simulink model "bldc_normal"  (R2020b)
settings: Solver=ode23t  StartTime=0  StopTime=500  FixedStep=Ts  MaxStep=1e-6  RelTol=1e-6  AbsTol=1e-6  EnableMultiTasking=on
PreLoadFcn:
  | assignin('base','Ts',[5e-6])
values from neighbouring files (symbols this model uses):
  N = speed.signals.values    [code.m]
libraries: powerlib x14
Description:
  | This demonstration illustrates use of the BLDC in a closed-loop
  | speed and voltage control on a 1 kW, 3000 rpm industrial motor
  | 
  | 
  | Copyright 2008-2010 The MathWorks, Inc.
settings Model: ExtModeAutoUpdateStatusClock=off  Creator=MathWorks  LastModifiedBy=yuvan
settings SolverCC: AutoScaleAbsTol=off  ZeroCrossControl=DisableAll  ZeroCrossAlgorithm=Adaptive
settings DataIOCC: LimitDataPoints=on  SaveFormat=Array  SignalLoggingSaveFormat=ModelDataLogs  ReturnWorkspaceOutputs=off  SignalLoggingName=sigsOut
settings OptimizationCC: ExpressionDepthLimit=2147483647  InitFltsAndDblsToZero=on  LifeSpan=inf
settings DebuggingCC: UnderspecifiedInitializationDetection=Classic  MergeDetectMultiDrivingBlocksExec=none  SignalResolutionControl=TryResolveAllWithWarning  MultiTaskDSMMsg=warning  MultiTaskCondExecSysMsg=none  FcnCallInpInsideContextMsg=warning  StateNameClashWarn=warning  SFUnexpectedBacktrackingDiag=warning  SFNoUnconditionalDefaultTransitionDiag=warning  SFExecutionAtInitializationDiag=none  ArithmeticOperatorsInVariantConditions=warning
settings HardwareCC: ProdBitPerPointer=32  ProdBitPerSizeT=32  ProdBitPerPtrDiffT=32  ProdLargestAtomicFloat=None  ProdIntDivRoundTo=Undefined  ProdEndianess=Unspecified  ProdWordSize=32  ProdHWDeviceType=32-bit Generic  TargetUnknown=on
settings ModelReferenceCC: PropagateSignalLabelsOutOfModel=off
settings SFSimCC: SimUseLocalCustomCode=off  CustomCodeUndefinedFunction=UseInterfaceOnly
settings RTWCC: RTWUseLocalCustomCode=off
settings CodeAppCC: StateflowObjectComments=on
settings GRTTargetCC: TargetLangStandard=C89/C90 (ANSI)  CombineOutputUpdateFcns=off  GRTInterface=on
settings ConfigComp: CovMetricSettings=dw  CovSaveCumulativeToWorkspaceVar=on  CovSaveSingleToWorkspaceVar=on  CovExternalEMLEnable=off
settings SimscapeCC: SimscapeNormalizeSystem=off

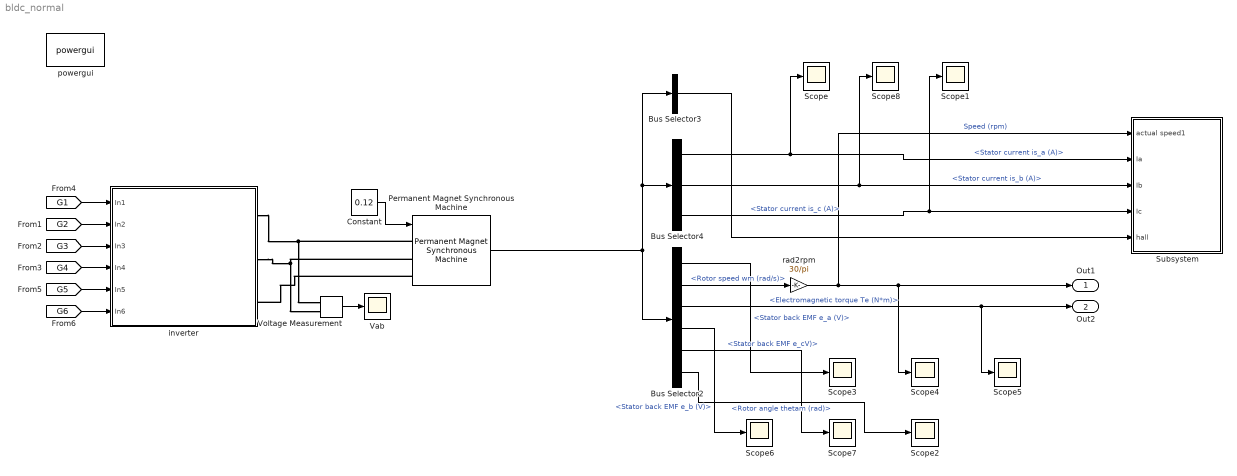
== system bldc_normal ==
  Bus Selector2 : BusSelector  OutputSignals=Stator back EMF e_a (V),Rotor speed wm (rad/s),Electromagnetic torque Te (N*m),Stator back EMF e_b (V),Stator back EMF e_cV),Rotor angle thetam (rad)
  Bus Selector3 : BusSelector  OutputSignals=Hall effect signal h_a,Hall effect signal h_b,Hall effect signal h_c  OutputAsBus=on
  Bus Selector4 : BusSelector  OutputSignals=Stator current is_a (A),Stator current is_b (A),Stator current is_c (A)
  Constant : Constant  Value=0.12
  Permanent Magnet Synchronous Machine : powerlib/Machines/Permanent Magnet Synchronous Machine  NbPhases=3  FluxDistribution=Trapezoidal  RotorType=Round  MechanicalLoad=Torque Tm  PresetModel=No  ShowDetailedParameters=on  MeasurementBus=off  Resistance=0.18  Inductance=0.000835  dqInductances=[8.5e-3,8.5e-3]  La=0.000835  MachineConstant=Torque Constant (N.m / A_peak)  Flux=0.015  VoltageCst=12.5664  TorqueCst=0.12  Flat=120  Mechanical=[0.000621417 0.000303448 4]  PolePairs=4  InitialConditions=[0,0, 0,0]  InitialConditions5ph=[0 0 0 0 0 0]  RefAngle=90 degrees behind phase A axis (modified Park)  IterativeDiscreteModel=Trapezoidal non iterative  TsBlock=-1  TsPowergui=0
  Scope{,1..8} (9 alike) : Scope
  Subsystem : Subsystem
  Vab : Scope
  Voltage Measurement : powerlib/Measurements/Voltage Measurement  PhasorSimulation=off  OutputType=Complex  PSBequivalent=0
  inverter : Subsystem
  powergui : powerlib/powergui  Priority=1  SimulationMode=Continuous  SampleTime=5e-6  frequency=60  Iterations=50  frequencyindice=0  Pbase=100e6  ErrMax=1e-4  UnitsV=kV  UnitsW=MW  buscounter=0  FunctionMessages=off  echomessages=off  EnableUseOfTLC=off  CurrentSourceSwitches=on  DisableSnubberDevices=off  DisableRonSwitches=off  DisableVfSwitches=off  DisplayEquations=off  AutomaticDiscreteSolvers=off  SolverType=Tustin/Backward Euler (TBE)  Interpol=off  ExternalGateDelay=off  methode=off  Ts=100  x0status=blocks  SPID=off  SwTol=0  HookPort=off  NonlinearTolerance=1e-4  nMaxIteration=100  ContinueOnMaxIteration=off  RestoreLinks=warning  ResistiveCurrentMeasurement=off  Frange=[0:2:500]  Ylog=off  Xlog=on  ShowGrid=off  save=off  variable=ZData  structure=0  ZoomFFT=off  StartTime=0.0  cycles=1  DisplayStyle=1  fundamental=60  FreqAxis=off  MaxFrequency=1000  frequencyindicesteady=1  RmsSteady=1  display=off
  rad2rpm : Gain  Gain=30/pi
  Out1 : Outport  VectorParamsAs1DForOutWhenUnconnected=off
  Out2 : Outport  Port=2  VectorParamsAs1DForOutWhenUnconnected=off
  wires:
  Constant/1 -> Permanent Magnet Synchronous Machine/1
  Voltage Measurement/1 -> Vab/1
  Permanent Magnet Synchronous Machine/1 -> Bus Selector3/1, Bus Selector4/1, Bus Selector2/1
  Bus Selector2/3 -> Scope5/1, Out2/1  "<Electromagnetic torque Te (N*m)>"
  rad2rpm/1 -> Subsystem/1(actual speed1), Scope4/1, Out1/1  "Speed (rpm)"
  Bus Selector2/2 -> rad2rpm/1  "<Rotor speed wm (rad/s)>"
  Bus Selector3/1 -> Subsystem/5(hall)
  Bus Selector4/1 -> Scope/1, Subsystem/2(Ia)  "<Stator current is_a (A)>"
  Bus Selector4/2 -> Scope8/1, Subsystem/3(Ib)  "<Stator current is_b (A)>"
  Bus Selector4/3 -> Scope1/1, Subsystem/4(Ic)  "<Stator current is_c (A)>"
  [G1] -> inverter/1(In1)
  [G2] -> inverter/2(In2)
  [G3] -> inverter/3(In3)
  [G4] -> inverter/4(In4)
  [G5] -> inverter/5(In5)
  [G6] -> inverter/6(In6)
  Bus Selector2/4 -> Scope6/1  "<Stator back EMF e_b (V)>"
  Bus Selector2/5 -> Scope7/1  "<Stator back EMF e_cV)>"
  Bus Selector2/6 -> Scope2/1  "<Rotor angle thetam (rad)>"
  Bus Selector2/1 -> Scope3/1  "<Stator back EMF e_a (V)>"
  connections:
  Permanent Magnet Synchronous Machine/LConn3 -- inverter/RConn3
  inverter/RConn1 -- Permanent Magnet Synchronous Machine/LConn1 -- Voltage Measurement/LConn1
  inverter/RConn2 -- Permanent Magnet Synchronous Machine/LConn2 -- Voltage Measurement/LConn2

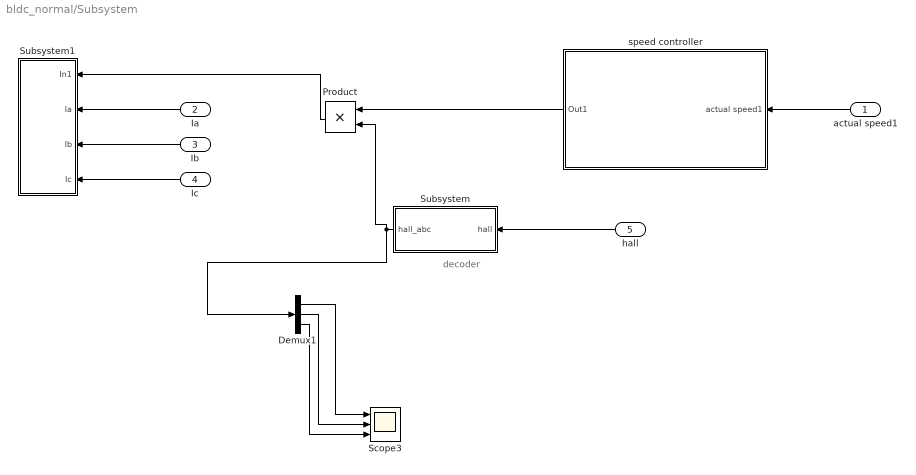
== system bldc_normal/Subsystem ==
  note: decoder
  actual speed1 : Inport
  Ia : Inport  Port=2
  Ib : Inport  Port=3
  Ic : Inport  Port=4
  hall : Inport  Port=5
  Demux1 : Demux  Outputs=3
  Product : Product
  Scope3 : Scope  NumInputPorts=3
  Subsystem : Subsystem
  Subsystem1 : Subsystem
  speed controller : Subsystem
  wires:
  speed controller/1(Out1) -> Product/1
  actual speed1/1 -> speed controller/1(actual speed1)
  Ib/1 -> Subsystem1/3(Ib)
  Ic/1 -> Subsystem1/4(Ic)
  Ia/1 -> Subsystem1/2(Ia)
  Product/1 -> Subsystem1/1(In1)
  Subsystem/1(hall_abc) -> Product/2, Demux1/1
  hall/1 -> Subsystem/1(hall)
  Demux1/1 -> Scope3/1
  Demux1/2 -> Scope3/2
  Demux1/3 -> Scope3/3

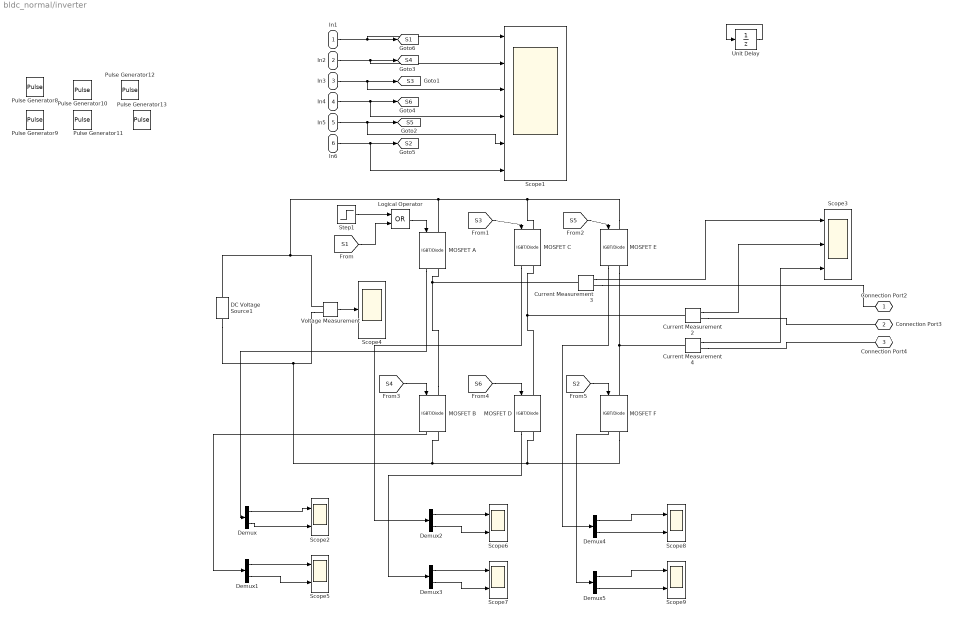
== system bldc_normal/inverter ==
  In1 : Inport
  In2 : Inport  Port=2
  In3 : Inport  Port=3
  In4 : Inport  Port=4
  In5 : Inport  Port=5
  In6 : Inport  Port=6
  Current Measurement2 : powerlib/Measurements/Current Measurement  PhasorSimulation=off  OutputType=Complex  PSBequivalent=0
  Current Measurement3 : powerlib/Measurements/Current Measurement  PhasorSimulation=off  OutputType=Complex  PSBequivalent=0
  Current Measurement4 : powerlib/Measurements/Current Measurement  PhasorSimulation=off  OutputType=Complex  PSBequivalent=0
  DC Voltage Source1 : powerlib/Electrical Sources/DC Voltage Source  Amplitude=48  Measurements=None
  Demux{,1..5} (6 alike) : Demux  Outputs=2
  Logical Operator : Logic  Operator=OR  AllPortsSameDT=off  OutDataTypeStr=boolean
  MOSFET A : powerlib/Power Electronics/IGBT//Diode  Ron=1e-3  Rs=500  Cs=1e-3  Measurements=on
  MOSFET B : powerlib/Power Electronics/IGBT//Diode  Ron=1e-3  Rs=500  Cs=1e-3  Measurements=on
  MOSFET C : powerlib/Power Electronics/IGBT//Diode  Ron=1e-3  Rs=500  Cs=1e-3  Measurements=on
  MOSFET D : powerlib/Power Electronics/IGBT//Diode  Ron=1e-3  Rs=500  Cs=1e-3  Measurements=on
  MOSFET E : powerlib/Power Electronics/IGBT//Diode  Ron=1e-3  Rs=500  Cs=1e-3  Measurements=on
  MOSFET F : powerlib/Power Electronics/IGBT//Diode  Ron=1e-3  Rs=500  Cs=1e-3  Measurements=on
  Pulse Generator10 : DiscretePulseGenerator  PulseType=Time based  Period=0.02  PulseWidth=50  PhaseDelay=6.67e-3
  Pulse Generator11 : DiscretePulseGenerator  PulseType=Time based  Period=0.02  PulseWidth=50  PhaseDelay=16.67e-3
  Pulse Generator12 : DiscretePulseGenerator  PulseType=Time based  Period=0.02  PulseWidth=50  PhaseDelay=13.33e-3
  Pulse Generator13 : DiscretePulseGenerator  PulseType=Time based  Period=0.02  PulseWidth=50  PhaseDelay=3.33e-3
  Pulse Generator8 : DiscretePulseGenerator  PulseType=Time based  Period=0.02  PulseWidth=50
  Pulse Generator9 : DiscretePulseGenerator  PulseType=Time based  Period=0.02  PulseWidth=50  PhaseDelay=0.01
  Scope1 : Scope  NumInputPorts=6
  Scope{2,5..9} (6 alike) : Scope  NumInputPorts=2
  Scope3 : Scope  NumInputPorts=3
  Scope4 : Scope
  Step1 : Step  Time=0.05  SampleTime=0
  Unit Delay : UnitDelay  SampleTime=1/40e-7  HasFrameUpgradeWarning=on
  Voltage Measurement : powerlib/Measurements/Voltage Measurement  PhasorSimulation=off  OutputType=Complex  PSBequivalent=0
  Connection Port2 : PMIOPort  Tag=PMCPort  Side=Right
  Connection Port3 : PMIOPort  Tag=PMCPort  Port=2  Side=Right
  Connection Port4 : PMIOPort  Tag=PMCPort  Port=3  Side=Right
  tag scope: S1=global, S2=global, S3=global, S4=global, S5=global, S6=global
  wires:
  Unit Delay/1 -> Unit Delay/1
  [S3] -> MOSFET C/1
  [S4] -> MOSFET B/1
  [S6] -> MOSFET D/1
  [S2] -> MOSFET F/1
  [S5] -> MOSFET E/1
  Voltage Measurement/1 -> Scope4/1
  Current Measurement3/1 -> Scope3/1
  In1/1 -> [S1], Scope1/1
  In2/1 -> [S4], Scope1/2
  In6/1 -> [S2], Scope1/6
  In3/1 -> [S3], Scope1/3
  In4/1 -> [S6], Scope1/4
  In5/1 -> [S5], Scope1/5
  Current Measurement2/1 -> Scope3/2
  Current Measurement4/1 -> Scope3/3
  MOSFET A/1 -> Demux/1
  Demux/1 -> Scope2/1
  Demux/2 -> Scope2/2
  MOSFET B/1 -> Demux1/1
  MOSFET C/1 -> Demux2/1
  MOSFET D/1 -> Demux3/1
  MOSFET E/1 -> Demux4/1
  MOSFET F/1 -> Demux5/1
  Demux2/1 -> Scope6/1
  Demux2/2 -> Scope6/2
  Demux3/1 -> Scope7/1
  Demux3/2 -> Scope7/2
  Demux4/1 -> Scope8/1
  Demux4/2 -> Scope8/2
  Demux5/1 -> Scope9/1
  Demux5/2 -> Scope9/2
  Demux1/1 -> Scope5/1
  Demux1/2 -> Scope5/2
  Logical Operator/1 -> MOSFET A/1
  Step1/1 -> Logical Operator/1
  [S1] -> Logical Operator/2
  connections:
  Voltage Measurement/LConn2 -- MOSFET F/RConn1 -- MOSFET D/RConn1 -- MOSFET B/RConn1 -- DC Voltage Source1/LConn1
  MOSFET B/LConn1 -- MOSFET A/RConn1 -- Current Measurement3/LConn1
  MOSFET D/LConn1 -- MOSFET C/RConn1 -- Current Measurement2/LConn1
  MOSFET E/RConn1 -- MOSFET F/LConn1 -- Current Measurement4/LConn1
  Current Measurement3/RConn1 -- Connection Port2/RConn1
  Current Measurement2/RConn1 -- Connection Port3/RConn1
  Current Measurement4/RConn1 -- Connection Port4/RConn1
  MOSFET E/LConn1 -- Voltage Measurement/LConn1 -- DC Voltage Source1/RConn1 -- MOSFET A/LConn1 -- MOSFET C/LConn1

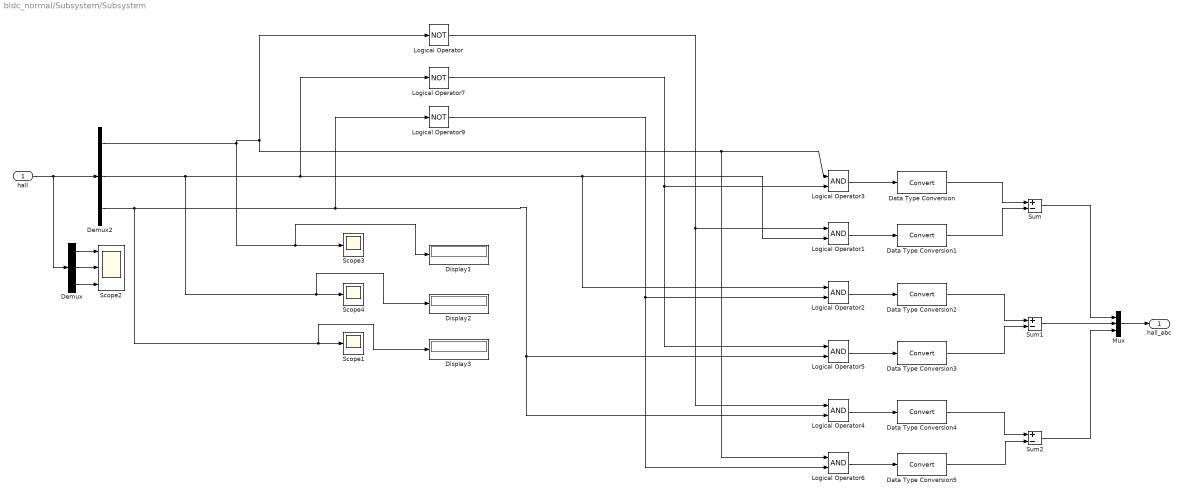
== system bldc_normal/Subsystem/Subsystem ==
  hall : Inport
  Data Type Conversion{,1..5} (6 alike) : DataTypeConversion
  Demux : Demux  Outputs=3
  Demux2 : Demux  Outputs=3
  Display1 : Display
  Display2 : Display
  Display3 : Display
  Logical Operator : Logic  Operator=NOT  AllPortsSameDT=off  OutDataTypeStr=boolean
  Logical Operator{1..6} (6 alike) : Logic  AllPortsSameDT=off  OutDataTypeStr=boolean
  Logical Operator7 : Logic  Operator=NOT  AllPortsSameDT=off  OutDataTypeStr=boolean
  Logical Operator9 : Logic  Operator=NOT  AllPortsSameDT=off  OutDataTypeStr=boolean
  Mux : Mux  Inputs=3
  Scope1 : Scope
  Scope2 : Scope  NumInputPorts=3
  Scope3 : Scope
  Scope4 : Scope
  Sum : Sum  Inputs=+-
  Sum1 : Sum  Inputs=+-
  Sum2 : Sum  Inputs=+-
  hall_abc : Outport  VectorParamsAs1DForOutWhenUnconnected=off
  wires:
  Logical Operator3/1 -> Data Type Conversion/1
  Logical Operator1/1 -> Data Type Conversion1/1
  Data Type Conversion1/1 -> Sum/2
  Logical Operator2/1 -> Data Type Conversion2/1
  Logical Operator5/1 -> Data Type Conversion3/1
  Data Type Conversion2/1 -> Sum1/1
  Data Type Conversion3/1 -> Sum1/2
  Sum1/1 -> Mux/2
  Logical Operator4/1 -> Data Type Conversion4/1
  Logical Operator6/1 -> Data Type Conversion5/1
  Data Type Conversion4/1 -> Sum2/1
  Data Type Conversion5/1 -> Sum2/2
  Sum2/1 -> Mux/3
  Mux/1 -> hall_abc/1
  Logical Operator7/1 -> Logical Operator5/1, Logical Operator3/2
  Logical Operator/1 -> Logical Operator4/1, Logical Operator1/1
  Logical Operator9/1 -> Logical Operator6/2, Logical Operator2/2
  Data Type Conversion/1 -> Sum/1
  Sum/1 -> Mux/1
  Demux2/1 -> Logical Operator6/1, Logical Operator3/1, Logical Operator/1, Display1/1, Scope3/1
  Demux2/2 -> Display2/1, Scope4/1, Logical Operator7/1, Logical Operator2/1, Logical Operator1/2
  Demux2/3 -> Scope1/1, Display3/1, Logical Operator9/1, Logical Operator4/2, Logical Operator5/2
  Demux/2 -> Scope2/2
  Demux/1 -> Scope2/1
  hall/1 -> Demux/1, Demux2/1
  Demux/3 -> Scope2/3

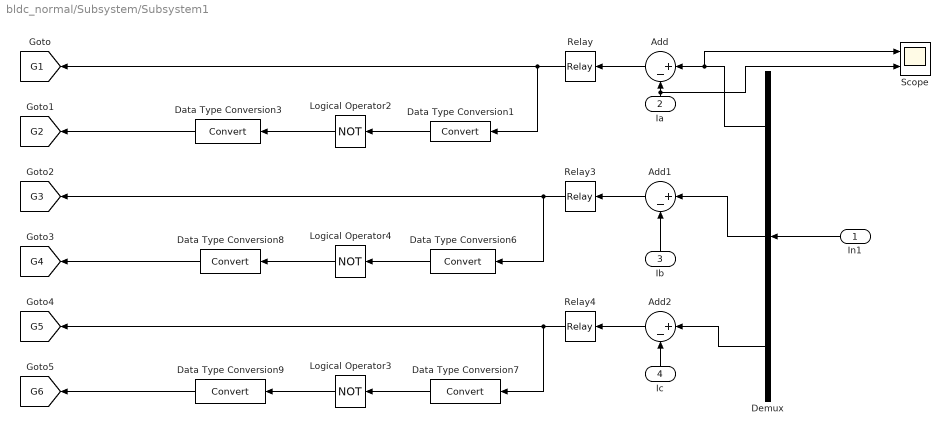
== system bldc_normal/Subsystem/Subsystem1 ==
  In1 : Inport
  Ia : Inport  Port=2
  Ib : Inport  Port=3
  Ic : Inport  Port=4
  Add : Sum  Inputs=|+-
  Add1 : Sum  Inputs=|+-
  Add2 : Sum  Inputs=|+-
  Data Type Conversion{1,3,6..9} (6 alike) : DataTypeConversion
  Demux : Demux  Outputs=3
  Logical Operator2 : Logic  Operator=NOT  AllPortsSameDT=off  OutDataTypeStr=boolean
  Logical Operator3 : Logic  Operator=NOT  AllPortsSameDT=off  OutDataTypeStr=boolean
  Logical Operator4 : Logic  Operator=NOT  AllPortsSameDT=off  OutDataTypeStr=boolean
  Relay : Relay  OnSwitchValue=0.005  OffSwitchValue=-0.005
  Relay3 : Relay  OnSwitchValue=0.05  OffSwitchValue=-0.05
  Relay4 : Relay  OnSwitchValue=0.05  OffSwitchValue=-0.05
  Scope : Scope  NumInputPorts=2
  tag scope: G1=global, G2=global, G3=global, G4=global, G5=global, G6=global
  wires:
  Data Type Conversion8/1 -> [G4]
  Relay4/1 -> [G5], Data Type Conversion7/1
  Relay3/1 -> [G3], Data Type Conversion6/1
  Data Type Conversion3/1 -> [G2]
  Data Type Conversion6/1 -> Logical Operator4/1
  Logical Operator4/1 -> Data Type Conversion8/1
  Logical Operator3/1 -> Data Type Conversion9/1
  Data Type Conversion1/1 -> Logical Operator2/1
  Relay/1 -> [G1], Data Type Conversion1/1
  Logical Operator2/1 -> Data Type Conversion3/1
  Data Type Conversion9/1 -> [G6]
  Data Type Conversion7/1 -> Logical Operator3/1
  Ia/1 -> Scope/2, Add/2
  Ic/1 -> Add2/2
  Demux/2 -> Add1/1
  Demux/3 -> Add2/1
  In1/1 -> Demux/1
  Demux/1 -> Scope/1, Add/1
  Add/1 -> Relay/1
  Ib/1 -> Add1/2
  Add1/1 -> Relay3/1
  Add2/1 -> Relay4/1

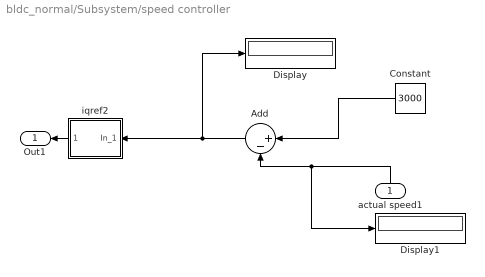
== system bldc_normal/Subsystem/speed controller ==
  actual speed1 : Inport
  Add : Sum  Inputs=|+-
  Constant : Constant  Value=3000
  Display : Display
  Display1 : Display
  iqref2 : Subsystem  mask(PI Controller){I=5, P=10, sat=[-50, 50]}
      mask prompts: I "Integral"; P "Proportional:"; sat "Minimum and maximum outputs:"
      mask init:
      | min=sat(1);max=sat(2);
      mask Display: disp('PI')
  Out1 : Outport  VectorParamsAs1DForOutWhenUnconnected=off
  wires:
  iqref2/1(Out_1) -> Out1/1
  actual speed1/1 -> Add/2, Display1/1
  Constant/1 -> Add/1
  Add/1 -> Display/1, iqref2/1(In_1)

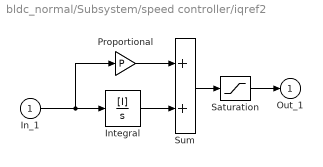
== system bldc_normal/Subsystem/speed controller/iqref2 ==
  In_1 : Inport
  Integral : TransferFcn  Numerator=[I]  Denominator=[1 0]
  Proportional : Gain  Gain=P  SaturateOnIntegerOverflow=on  OutDataTypeStr=Inherit: Same as input  ParamDataTypeStr=Inherit: Same as input
  Saturation : Saturate  UpperLimit=max  LowerLimit=min
  Sum : Sum  InputSameDT=on  SaturateOnIntegerOverflow=on  OutDataTypeStr=Inherit: Same as first input
  Out_1 : Outport  InitialOutput=0  VectorParamsAs1DForOutWhenUnconnected=off
  wires:
  Integral/1 -> Sum/2
  In_1/1 -> Integral/1, Proportional/1
  Proportional/1 -> Sum/1
  Sum/1 -> Saturation/1
  Saturation/1 -> Out_1/1
